simulink library "kinematics"  (R2021b)
settings: Solver=VariableStepAuto  StartTime=0.0  StopTime=10.0  RelTol=1e-3
settings Model: Creator=Nikita  LastModifiedBy=Nikita
settings SolverCC: AlgebraicLoopSolver=TrustRegion
settings DebuggingCC: SFMachineParentedDataDiag=warning

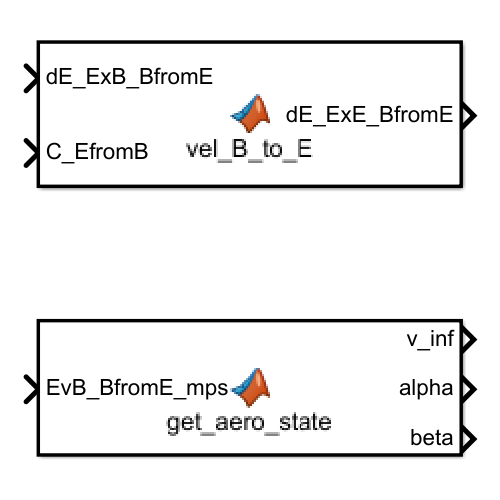
[thumbnail: Simulink's stored preview of the top-level diagram]
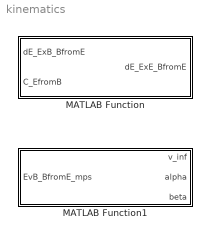
== system kinematics ==
  MATLAB Function : MATLAB Function  TreatAsAtomicUnit=on
  MATLAB Function1 : MATLAB Function  TreatAsAtomicUnit=on

== matlab function kinematics/MATLAB Function ==
  data: dE_ExB_BfromE input; dE_ExE_BfromE output; C_EfromB input
% This function converts the time rate of change in ECEF frame of the
% position vector of the body wrt the Earth in the ECEF frame and the Body
% coordinate system to its counterpart in the ECEF coordinate system.
%
% Not sure about the naming convention, but this does include all needed
% info
function dE_ExE_BfromE = vel_B_to_E(dE_ExB_BfromE, C_EfromB)

dE_ExE_BfromE = C_EfromB*dE_ExB_BfromE;

== matlab function kinematics/MATLAB Function1 ==
  data: EvB_BfromE_mps input; v_inf output; alpha output; beta output
function [v_inf, alpha, beta] = get_aero_state(EvB_BfromE_mps)

v_inf   = norm(EvB_BfromE_mps);
alpha   = atan2(EvB_BfromE_mps(3), EvB_BfromE_mps(1));
beta    = atan2(EvB_BfromE_mps(2), v_inf);
